simulink model "IIR"  (R2013a)
settings: Solver=ode45  StartTime=0.0  StopTime=0.5  RelTol=1e-5
settings Model: Creator=Max Simmonds  LastModifiedBy=Max Simmonds

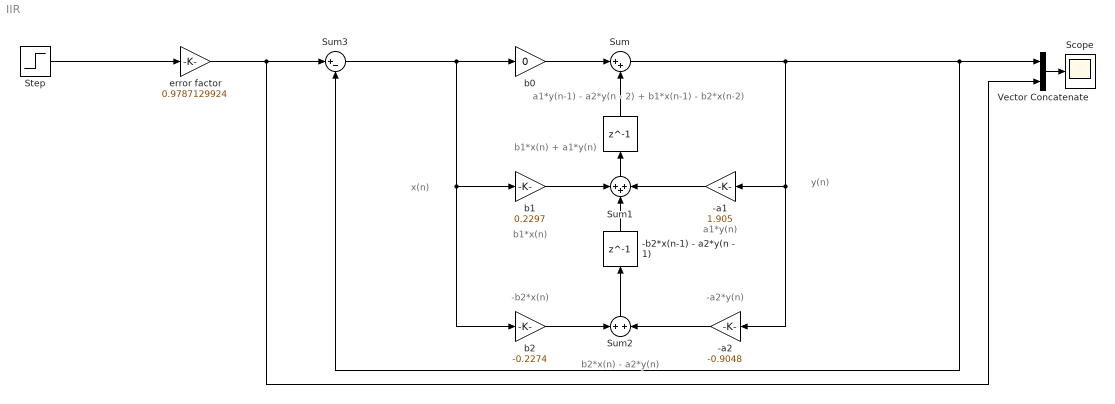
== system IIR ==
  note: a1*y(n-1) - a2*y(n - 2) + b1*x(n-1) - b2*x(n-2)
  note: y(n)
  note: a1*y(n)
  note: -a2*y(n)
  note: b2*x(n) - a2*y(n)
  note: -b2*x(n)
  note: b1*x(n) + a1*y(n)
  note: x(n)
  note: b1*x(n)
  " " : Delay  DelayLength=1  InitialCondition=0  SampleTime=0.000001
  -a1 : Gain  Gain=1.905
  -a2 : Gain  Gain=-0.9048
  -b2*x(n-1) - a2*y(n - 1) : Delay  DelayLength=1  InitialCondition=0  SampleTime=0.000001
  Scope : Scope
      settings: TimeRange=0.002144777321648694  YMin=0  YMax=1.225021720243266
  Step : Step  Time=0.25  SampleTime=0
  Sum : Sum  Inputs=|++  SampleTime=0.000001
  Sum1 : Sum  Inputs=+++  SampleTime=0.000001
  Sum2 : Sum  SampleTime=0.000001
  Sum3 : Sum  Inputs=|+-  SampleTime=0.000001
  Vector Concatenate : Concatenate
  "b0 " : Gain  Gain=0
  b1 : Gain  Gain=0.2297
  b2 : Gain  Gain=-0.2274
  error factor : Gain  Gain=0.9787129924
  wires:
  " "/1 -> Sum/2
  -b2*x(n-1) - a2*y(n - 1)/1 -> Sum1/2
  Sum1/1 -> " "/1
  Sum2/1 -> -b2*x(n-1) - a2*y(n - 1)/1
  b1/1 -> Sum1/1
  "b0 "/1 -> Sum/1
  b2/1 -> Sum2/1
  -a1/1 -> Sum1/3
  -a2/1 -> Sum2/2
  Sum/1 -> Sum3/2, Vector Concatenate/1, -a2/1, -a1/1
  Vector Concatenate/1 -> Scope/1
  Sum3/1 -> b2/1, b1/1, "b0 "/1
  error factor/1 -> Vector Concatenate/2, Sum3/1
  Step/1 -> error factor/1
